simulink model "exFlexOP"  (R2025a)
settings: Solver=VariableStepAuto  StartTime=0.0  StopTime=10.0  RelTol=1e-3
values from neighbouring files (symbols this model uses):
  b = 1.0    [exFlexOp_dd.sldd]    (also in massSpringDamperDD.sldd = 100.0)
undefined symbols (not defined in the file or in its folder): magnitude
settings Model: DataDictionary=exFlexOp_dd.sldd  Creator=grouleau  LastModifiedBy=grouleau

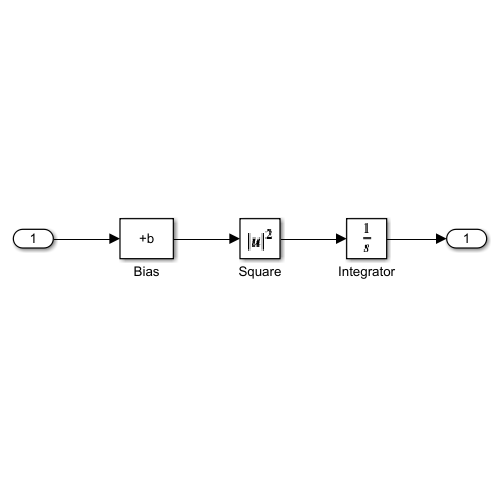
[thumbnail: Simulink's stored preview of the top-level diagram]
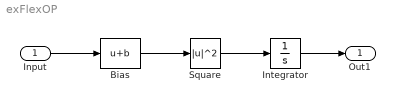
== system exFlexOP ==
  Input : Inport
  Bias : Bias  Bias=b  SaturateOnIntegerOverflow=off
  Integrator : Integrator
  Square : Math  Operator=magnitude^2
  Out1 : Outport
  wires:
  Input/1 -> Bias/1
  Bias/1 -> Square/1
  Integrator/1 -> Out1/1
  Square/1 -> Integrator/1
